simulink model "top_level_arch"  (R2025b)
settings: Solver=VariableStepAuto  StartTime=0.0  StopTime=10.0  RelTol=1e-3
undefined symbols (not defined in the file): D, L
(part 1 of 2)
settings Model: Creator=andgo  LastModifiedBy=andgo

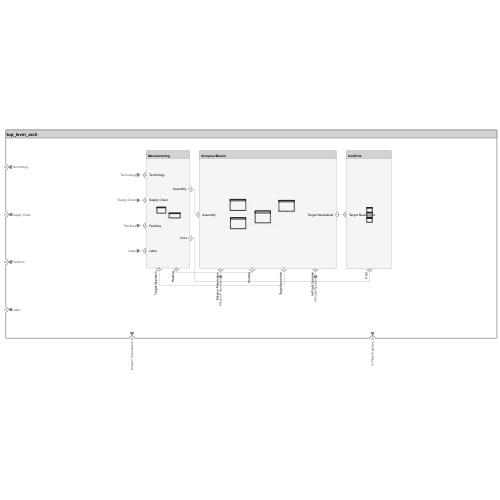
[thumbnail: Simulink's stored preview of the top-level diagram]
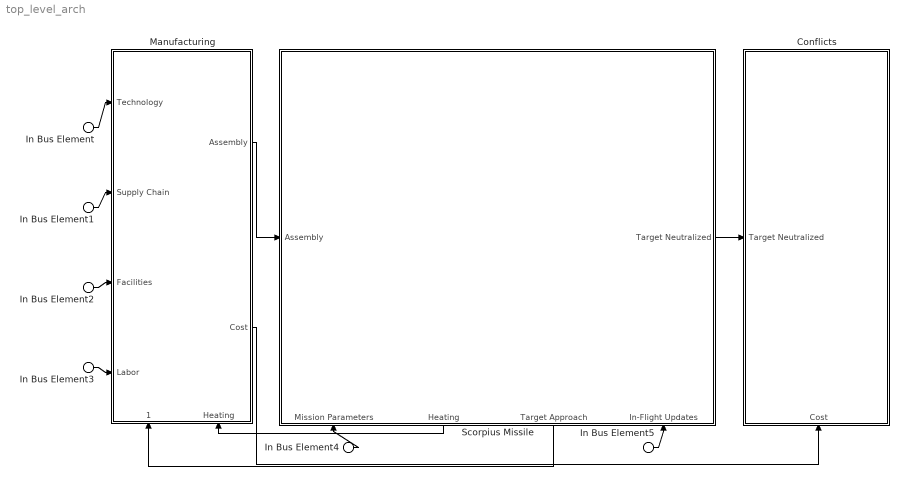
== system top_level_arch ==
  In Bus Element : Inport  PortName=Technology
  In Bus Element1 : Inport  Port=2  PortName=Supply Chain
  In Bus Element2 : Inport  Port=3  PortName=Facilities
  In Bus Element3 : Inport  Port=4  PortName=Labor
  In Bus Element4 : Inport  Port=5  PortName=Mission Parameters
  In Bus Element5 : Inport  Port=6  PortName=In-Flight Updates
  Conflicts : Subsystem
      settings: PortSchema="{\"entries\":[{\"content\":{\"headerSize\":26,\"margin\":15,\"minimumSpacing\":25,\"sides\":[{\"content\":{\"connectorIds\":[\"In2\"]},\"type\":\"ConnectorPlacement.EquallySpacedRectSide\",\"uuid\":\"acffec25-5f7e-46a6-bfc3-7ef631e1638e\"},{\"content\":{\"side\":\"RIGHT\"},\"type\":\"ConnectorPlacement.EquallySpacedRectSide\",\"uuid\":\"2e9e2c31-11a0-4694-98ae-75af4a65f270\"},{\"content\":{\"side\":\"TOP\"},\"type\":\"ConnectorPlacement.EquallySpacedRectSide\",\"uuid\":\"496cd80b-0660-4c9b-9e86-ee3459eee66e\"},{\"content\":{\"connectorIds\":[\"In1\"],\"side\":\"BOTTOM\"},\"type\":\"ConnectorPlacement.EquallySpacedRectSide\",\"uuid\":\"28484b37-6b41-41f8-9797-a09ef52b9345\"}]},\"type\":\"ConnectorPlacement.EquallySpacedConnector\",\"uuid\":\"b09bcaf7-bc67-4c5f-bdb5-a74881794e47\"}],\"packageUris\":[\"http://schema.mathworks.com/mf0/Connector/R2020b\"],\"version\":\"1.0\"}"
  "Manufacturing " : Subsystem
      settings: PortSchema="{\"entries\":[{\"content\":{\"headerSize\":26,\"margin\":15,\"minimumSpacing\":25,\"sides\":[{\"content\":{\"connectorIds\":[\"In3\",\"In4\",\"In5\",\"In6\"]},\"type\":\"ConnectorPlacement.EquallySpacedRectSide\",\"uuid\":\"acffec25-5f7e-46a6-bfc3-7ef631e1638e\"},{\"content\":{\"connectorIds\":[\"Out1\",\"Out2\"],\"side\":\"RIGHT\"},\"type\":\"ConnectorPlacement.EquallySpacedRectSide\",\"uuid\":\"2e9e2c31-11a0-4694-98ae-75af4a65f270\"},{\"content\":{\"side\":\"TOP\"},\"type\":\"ConnectorPlacement.EquallySpacedRectSide\",\"uuid\":\"496cd80b-0660-4c9b-9e86-ee3459eee66e\"},{\"content\":{\"connectorIds\":[\"In1\",\"In2\"],\"side\":\"BOTTOM\"},\"type\":\"ConnectorPlacement.EquallySpacedRectSide\",\"uuid\":\"33532b3b-2f4b-483d-9516-7c4914e8cb27\"}]},\"type\":\"ConnectorPlacement.EquallySpacedConnector\",\"uuid\":\"b09bcaf7-bc67-4c5f-bdb5-a74881794e47\"}],\"packageUris\":[\"http://schema.mathworks.com/mf0/Connector/R2020b\"],\"version\":\"1.0\"}"
  Scorpius Missile : Subsystem
      settings: PortSchema="{\"entries\":[{\"content\":{\"headerSize\":26,\"margin\":15,\"minimumSpacing\":25,\"sides\":[{\"content\":{\"connectorIds\":[\"In3\"]},\"type\":\"ConnectorPlacement.EquallySpacedRectSide\",\"uuid\":\"acffec25-5f7e-46a6-bfc3-7ef631e1638e\"},{\"content\":{\"connectorIds\":[\"Out3\"],\"side\":\"RIGHT\"},\"type\":\"ConnectorPlacement.EquallySpacedRectSide\",\"uuid\":\"2e9e2c31-11a0-4694-98ae-75af4a65f270\"},{\"content\":{\"side\":\"TOP\"},\"type\":\"ConnectorPlacement.EquallySpacedRectSide\",\"uuid\":\"496cd80b-0660-4c9b-9e86-ee3459eee66e\"},{\"content\":{\"connectorIds\":[\"In1\",\"Out1\",\"Out2\",\"In2\"],\"side\":\"BOTTOM\"},\"type\":\"ConnectorPlacement.EquallySpacedRectSide\",\"uuid\":\"f0cf9de3-dec7-4c3c-836d-f09237c2a5d9\"}]},\"type\":\"ConnectorPlacement.EquallySpacedConnector\",\"uuid\":\"b09bcaf7-bc67-4c5f-bdb5-a74881794e47\"}],\"packageUris\":[\"http://schema.mathworks.com/mf0/Connector/R2020b\"],\"version\":\"1.0\"}"
  wires:
  Scorpius Missile/3(Target Neutralized) -> Conflicts/2(Target Neutralized)
  "Manufacturing "/1(Assembly) -> Scorpius Missile/3(Assembly)
  In Bus Element/1 -> "Manufacturing "/3(Technology)
  In Bus Element1/1 -> "Manufacturing "/4(Supply Chain)
  In Bus Element2/1 -> "Manufacturing "/5(Facilities)
  In Bus Element3/1 -> "Manufacturing "/6(Labor)
  In Bus Element4/1 -> Scorpius Missile/1(Mission Parameters)
  In Bus Element5/1 -> Scorpius Missile/2(In-Flight Updates)
  Scorpius Missile/1(Heating) -> "Manufacturing "/2(Heating)
  Scorpius Missile/2(Target Approach) -> "Manufacturing "/1(Target Approach)
  "Manufacturing "/2(Cost) -> Conflicts/1(Cost)

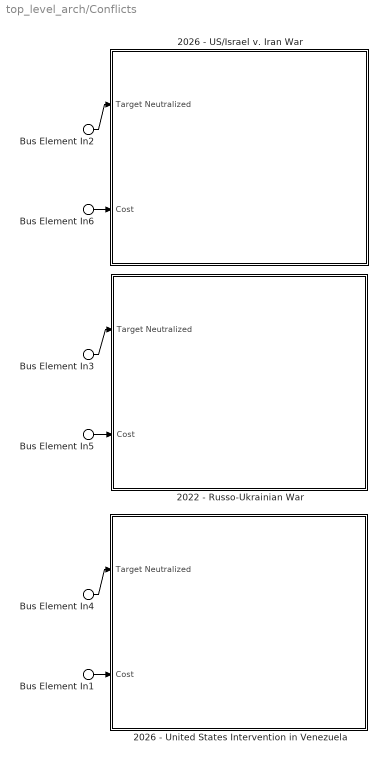
== system top_level_arch/Conflicts ==
  Bus Element In1 : Inport  PortName=Cost
  Bus Element In5 : Inport  PortName=Cost
  Bus Element In6 : Inport  PortName=Cost
  Bus Element In2 : Inport  Port=2  PortName=Target Neutralized
  Bus Element In3 : Inport  Port=2  PortName=Target Neutralized
  Bus Element In4 : Inport  Port=2  PortName=Target Neutralized
  2022 - Russo-Ukrainian War : Subsystem
      settings: PortSchema="{\"entries\":[{\"content\":{\"headerSize\":26,\"margin\":15,\"minimumSpacing\":25,\"sides\":[{\"content\":{\"connectorIds\":[\"In1\",\"In2\"]},\"type\":\"ConnectorPlacement.EquallySpacedRectSide\",\"uuid\":\"acffec25-5f7e-46a6-bfc3-7ef631e1638e\"},{\"content\":{\"side\":\"RIGHT\"},\"type\":\"ConnectorPlacement.EquallySpacedRectSide\",\"uuid\":\"2e9e2c31-11a0-4694-98ae-75af4a65f270\"},{\"content\":{\"side\":\"TOP\"},\"type\":\"ConnectorPlacement.EquallySpacedRectSide\",\"uuid\":\"496cd80b-0660-4c9b-9e86-ee3459eee66e\"}]},\"type\":\"ConnectorPlacement.EquallySpacedConnector\",\"uuid\":\"b09bcaf7-bc67-4c5f-bdb5-a74881794e47\"}],\"packageUris\":[\"http://schema.mathworks.com/mf0/Connector/R2020b\"],\"version\":\"1.0\"}"
  2026 - US/Israel v. Iran War : Subsystem
      settings: PortSchema="{\"entries\":[{\"content\":{\"headerSize\":26,\"margin\":15,\"minimumSpacing\":25,\"sides\":[{\"content\":{\"connectorIds\":[\"In1\",\"In2\"]},\"type\":\"ConnectorPlacement.EquallySpacedRectSide\",\"uuid\":\"acffec25-5f7e-46a6-bfc3-7ef631e1638e\"},{\"content\":{\"side\":\"RIGHT\"},\"type\":\"ConnectorPlacement.EquallySpacedRectSide\",\"uuid\":\"2e9e2c31-11a0-4694-98ae-75af4a65f270\"},{\"content\":{\"side\":\"TOP\"},\"type\":\"ConnectorPlacement.EquallySpacedRectSide\",\"uuid\":\"496cd80b-0660-4c9b-9e86-ee3459eee66e\"}]},\"type\":\"ConnectorPlacement.EquallySpacedConnector\",\"uuid\":\"b09bcaf7-bc67-4c5f-bdb5-a74881794e47\"}],\"packageUris\":[\"http://schema.mathworks.com/mf0/Connector/R2020b\"],\"version\":\"1.0\"}"
  2026 - United States Intervention in Venezuela : Subsystem
      settings: PortSchema="{\"entries\":[{\"content\":{\"headerSize\":26,\"margin\":15,\"minimumSpacing\":25,\"sides\":[{\"content\":{\"connectorIds\":[\"In1\",\"In2\"]},\"type\":\"ConnectorPlacement.EquallySpacedRectSide\",\"uuid\":\"acffec25-5f7e-46a6-bfc3-7ef631e1638e\"},{\"content\":{\"side\":\"RIGHT\"},\"type\":\"ConnectorPlacement.EquallySpacedRectSide\",\"uuid\":\"2e9e2c31-11a0-4694-98ae-75af4a65f270\"},{\"content\":{\"side\":\"TOP\"},\"type\":\"ConnectorPlacement.EquallySpacedRectSide\",\"uuid\":\"496cd80b-0660-4c9b-9e86-ee3459eee66e\"}]},\"type\":\"ConnectorPlacement.EquallySpacedConnector\",\"uuid\":\"b09bcaf7-bc67-4c5f-bdb5-a74881794e47\"}],\"packageUris\":[\"http://schema.mathworks.com/mf0/Connector/R2020b\"],\"version\":\"1.0\"}"
  wires:
  Bus Element In2/1 -> 2026 - US/Israel v. Iran War/1(Target Neutralized)
  Bus Element In3/1 -> 2022 - Russo-Ukrainian War/1(Target Neutralized)
  Bus Element In4/1 -> 2026 - United States Intervention in Venezuela/1(Target Neutralized)
  Bus Element In1/1 -> 2026 - United States Intervention in Venezuela/2(Cost)
  Bus Element In5/1 -> 2022 - Russo-Ukrainian War/2(Cost)
  Bus Element In6/1 -> 2026 - US/Israel v. Iran War/2(Cost)

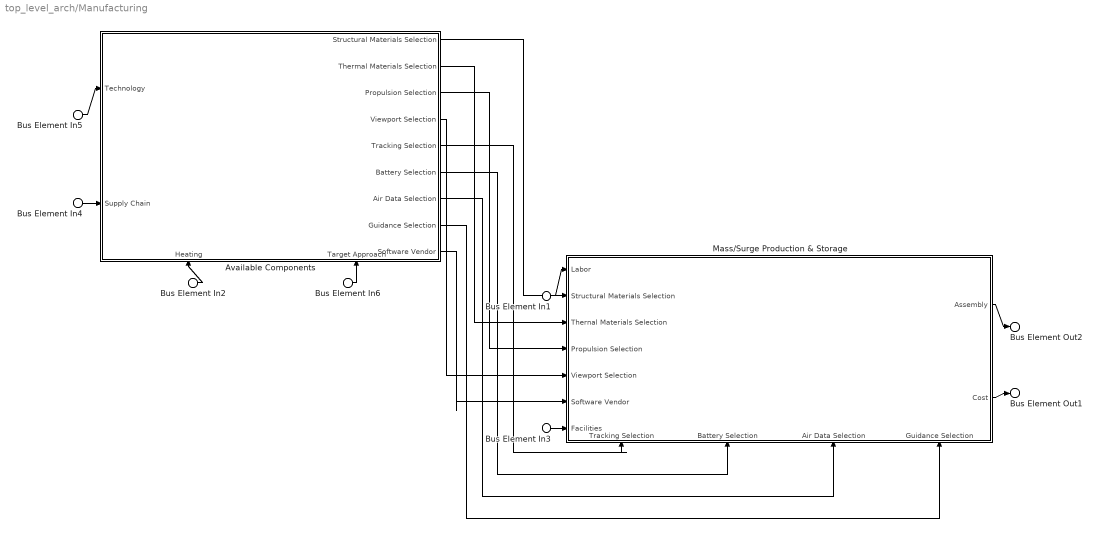
== system top_level_arch/Manufacturing  ==
  Bus Element In6 : Inport  PortName=Target Approach
  Bus Element In2 : Inport  Port=2  PortName=Heating
  Bus Element In5 : Inport  Port=3  PortName=Technology
  Bus Element In4 : Inport  Port=4  PortName=Supply Chain
  Bus Element In3 : Inport  Port=5  PortName=Facilities
  Bus Element In1 : Inport  Port=6  PortName=Labor
  Available Components : Subsystem
      settings: PortSchema="{\"entries\":[{\"content\":{\"headerSize\":26,\"margin\":15,\"minimumSpacing\":25,\"sides\":[{\"content\":{\"connectorIds\":[\"In3\",\"In4\"]},\"type\":\"ConnectorPlacement.EquallySpacedRectSide\",\"uuid\":\"acffec25-5f7e-46a6-bfc3-7ef631e1638e\"},{\"content\":{\"connectorIds\":[\"Out1\",\"Out2\",\"Out3\",\"Out4\",\"Out5\",\"Out6\",\"Out7\",\"Out8\",\"Out9\"],\"side\":\"RIGHT\"},\"type\":\"ConnectorPlacement.EquallySpacedRectSide\",\"uuid\":\"2e9e2c31-11a0-4694-98ae-75af4a65f270\"},{\"content\":{\"side\":\"TOP\"},\"type\":\"ConnectorPlacement.EquallySpacedRectSide\",\"uuid\":\"496cd80b-0660-4c9b-9e86-ee3459eee66e\"},{\"content\":{\"connectorIds\":[\"In1\",\"In2\"],\"side\":\"BOTTOM\"},\"type\":\"ConnectorPlacement.EquallySpacedRectSide\",\"uuid\":\"c248d288-a86e-4b39-8154-69971e55abdb\"}]},\"type\":\"ConnectorPlacement.EquallySpacedConnector\",\"uuid\":\"b09bcaf7-bc67-4c5f-bdb5-a74881794e47\"}],\"packageUris\":[\"http://schema.mathworks.com/mf0/Connector/R2020b\"],\"version\":\"1.0\"}"
  Mass/Surge Production & Storage : Subsystem
      settings: PortSchema="{\"entries\":[{\"content\":{\"headerSize\":26,\"margin\":15,\"minimumSpacing\":25,\"sides\":[{\"content\":{\"connectorIds\":[\"In6\",\"In7\",\"In8\",\"In9\",\"In5\",\"In10\",\"In11\"]},\"type\":\"ConnectorPlacement.EquallySpacedRectSide\",\"uuid\":\"0599d581-e05a-42f2-828a-909155d7b553\"},{\"content\":{\"connectorIds\":[\"Out1\",\"Out2\"],\"side\":\"RIGHT\"},\"type\":\"ConnectorPlacement.EquallySpacedRectSide\",\"uuid\":\"4f3684cd-c181-4c6b-8883-844072d01e34\"},{\"content\":{\"side\":\"TOP\"},\"type\":\"ConnectorPlacement.EquallySpacedRectSide\",\"uuid\":\"71c93445-b4b9-443f-b471-e335a3ed31ea\"},{\"content\":{\"connectorIds\":[\"In1\",\"In2\",\"In3\",\"In4\"],\"side\":\"BOTTOM\"},\"type\":\"ConnectorPlacement.EquallySpacedRectSide\",\"uuid\":\"e60e4bcf-0025-4c31-a0bb-395ca2e6fb9d\"}]},\"type\":\"ConnectorPlacement.EquallySpacedConnector\",\"uuid\":\"086a7661-e694-4344-b95d-ad0347bf3c95\"}],\"packageUris\":[\"http://schema.mathworks.com/mf0/Connector/R2020b\"],\"version\":\"1.0\"}"
  Bus Element Out2 : Outport  PortName=Assembly
  Bus Element Out1 : Outport  Port=2  PortName=Cost
  wires:
  Bus Element In1/1 -> Mass/Surge Production & Storage/6(Labor)
  Bus Element In3/1 -> Mass/Surge Production & Storage/11(Facilities)
  Available Components/1(Structural Materials Selection) -> Mass/Surge Production & Storage/7(Structural Materials Selection)
  Bus Element In5/1 -> Available Components/3(Technology)
  Bus Element In4/1 -> Available Components/4(Supply Chain)
  Mass/Surge Production & Storage/2(Cost) -> Bus Element Out1/1
  Mass/Surge Production & Storage/1(Assembly) -> Bus Element Out2/1
  Available Components/2(Thermal Materials Selection) -> Mass/Surge Production & Storage/8(Thernal Materials Selection)
  Available Components/3(Propulsion Selection) -> Mass/Surge Production & Storage/9(Propulsion Selection)
  Available Components/9(Software Vendor) -> Mass/Surge Production & Storage/10(Software Vendor)
  Available Components/5(Tracking Selection) -> Mass/Surge Production & Storage/1(Tracking Selection)
  Available Components/6(Battery Selection) -> Mass/Surge Production & Storage/2(Battery Selection)
  Available Components/7(Air Data Selection) -> Mass/Surge Production & Storage/3(Air Data Selection)
  Available Components/8(Guidance Selection) -> Mass/Surge Production & Storage/4(Guidance Selection)
  Bus Element In2/1 -> Available Components/1(Heating)
  Bus Element In6/1 -> Available Components/2(Target Approach)
  Available Components/4(Viewport Selection) -> Mass/Surge Production & Storage/5(Viewport Selection)

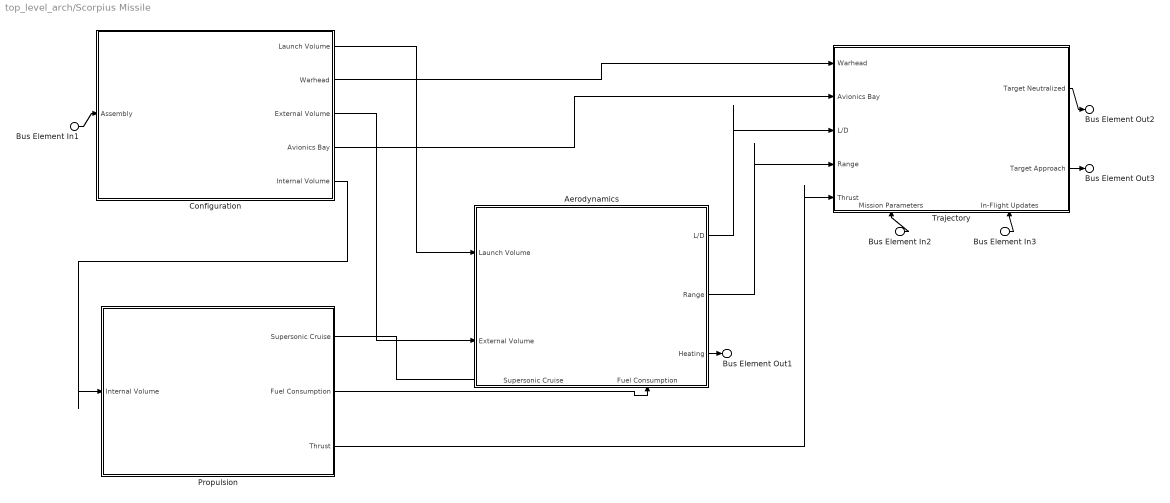
== system top_level_arch/Scorpius Missile ==
  Bus Element In2 : Inport  PortName=Mission Parameters
  Bus Element In3 : Inport  Port=2  PortName=In-Flight Updates
  Bus Element In1 : Inport  Port=3  PortName=Assembly
  Aerodynamics : Subsystem  Variant=on  VariantControlMode=label  LabelModeActiveChoice=true
      settings: PortSchema="{\"entries\":[{\"content\":{\"headerSize\":38,\"margin\":15,\"minimumSpacing\":25,\"sides\":[{\"content\":{\"connectorIds\":[\"In3\",\"In4\"]},\"type\":\"ConnectorPlacement.EquallySpacedRectSide\",\"uuid\":\"5f197e08-86ca-4cb0-8773-2eafa3be5f58\"},{\"content\":{\"connectorIds\":[\"Out2\",\"Out3\",\"Out1\"],\"side\":\"RIGHT\"},\"type\":\"ConnectorPlacement.EquallySpacedRectSide\",\"uuid\":\"8f6035a6-196b-436f-97c5-6c30a28d2ffa\"},{\"content\":{\"side\":\"TOP\"},\"type\":\"ConnectorPlacement.EquallySpacedRectSide\",\"uuid\":\"47fbcf31-f69d-4ec2-89cd-2bc4268e79ee\"},{\"content\":{\"connectorIds\":[\"In1\",\"In2\"],\"side\":\"BOTTOM\"},\"type\":\"ConnectorPlacement.EquallySpacedRectSide\",\"uuid\":\"4028af42-eefe-4e40-a537-59e66f9c77fb\"}]},\"type\":\"ConnectorPlacement.EquallySpacedConnector\",\"uuid\":\"7bd4d14b-9a13-45a8-b2b2-976268dd46fb\"}],\"packageUris\":[\"http://schema.mathworks.com/mf0/Connector/R2020b\"],\"version\":\"1.0\"}"
  Configuration : Subsystem
      settings: PortSchema="{\"entries\":[{\"content\":{\"headerSize\":26,\"margin\":15,\"minimumSpacing\":25,\"sides\":[{\"content\":{\"connectorIds\":[\"In1\"]},\"type\":\"ConnectorPlacement.EquallySpacedRectSide\",\"uuid\":\"32e1f4e9-0392-4c12-9305-55f9b62cf007\"},{\"content\":{\"connectorIds\":[\"Out3\",\"Out2\",\"Out5\",\"Out4\",\"Out1\"],\"side\":\"RIGHT\"},\"type\":\"ConnectorPlacement.EquallySpacedRectSide\",\"uuid\":\"8bf8c952-69c8-496e-947f-24d197d632d3\"},{\"content\":{\"side\":\"TOP\"},\"type\":\"ConnectorPlacement.EquallySpacedRectSide\",\"uuid\":\"adf3e777-baf5-48a6-a5b4-f0ede588bd33\"},{\"content\":{\"side\":\"BOTTOM\"},\"type\":\"ConnectorPlacement.EquallySpacedRectSide\",\"uuid\":\"91d27ee5-9ea1-4b68-a684-98df6014676a\"}]},\"type\":\"ConnectorPlacement.EquallySpacedConnector\",\"uuid\":\"9ec8f034-0877-461e-a570-0bf1a23861f1\"}],\"packageUris\":[\"http://schema.mathworks.com/mf0/Connector/R2020b\"],\"version\":\"1.0\"}"
  Propulsion : Subsystem  Description=|
      | Relevant Trade Study .m file listed in Stereotypes. 
      | Cannot link .m files directly.
      | Other teams encountered this issue as well.
      settings: PortSchema="{\"entries\":[{\"content\":{\"headerSize\":26,\"margin\":15,\"minimumSpacing\":25,\"sides\":[{\"content\":{\"connectorIds\":[\"In1\"]},\"type\":\"ConnectorPlacement.EquallySpacedRectSide\",\"uuid\":\"acffec25-5f7e-46a6-bfc3-7ef631e1638e\"},{\"content\":{\"connectorIds\":[\"Out1\",\"Out2\",\"Out3\"],\"side\":\"RIGHT\"},\"type\":\"ConnectorPlacement.EquallySpacedRectSide\",\"uuid\":\"2e9e2c31-11a0-4694-98ae-75af4a65f270\"},{\"content\":{\"side\":\"TOP\"},\"type\":\"ConnectorPlacement.EquallySpacedRectSide\",\"uuid\":\"496cd80b-0660-4c9b-9e86-ee3459eee66e\"}]},\"type\":\"ConnectorPlacement.EquallySpacedConnector\",\"uuid\":\"b09bcaf7-bc67-4c5f-bdb5-a74881794e47\"}],\"packageUris\":[\"http://schema.mathworks.com/mf0/Connector/R2020b\"],\"version\":\"1.0\"}"
  Trajectory : Subsystem  Description=|
      | Relevant Trade Study .m file listed in Stereotypes. 
      | Cannot link .m files directly.
      | Other teams encountered this issue as well.
      settings: PortSchema="{\"entries\":[{\"content\":{\"headerSize\":26,\"margin\":15,\"minimumSpacing\":25,\"sides\":[{\"content\":{\"connectorIds\":[\"In1\",\"In7\",\"In3\",\"In4\",\"In5\"]},\"type\":\"ConnectorPlacement.EquallySpacedRectSide\",\"uuid\":\"acffec25-5f7e-46a6-bfc3-7ef631e1638e\"},{\"content\":{\"connectorIds\":[\"Out1\",\"Out2\"],\"side\":\"RIGHT\"},\"type\":\"ConnectorPlacement.EquallySpacedRectSide\",\"uuid\":\"2e9e2c31-11a0-4694-98ae-75af4a65f270\"},{\"content\":{\"side\":\"TOP\"},\"type\":\"ConnectorPlacement.EquallySpacedRectSide\",\"uuid\":\"496cd80b-0660-4c9b-9e86-ee3459eee66e\"},{\"content\":{\"connectorIds\":[\"In2\",\"In6\"],\"side\":\"BOTTOM\"},\"type\":\"ConnectorPlacement.EquallySpacedRectSide\",\"uuid\":\"ff4f15f2-78c9-4b4d-8b3c-eee51a6070cf\"}]},\"type\":\"ConnectorPlacement.EquallySpacedConnector\",\"uuid\":\"b09bcaf7-bc67-4c5f-bdb5-a74881794e47\"}],\"packageUris\":[\"http://schema.mathworks.com/mf0/Connector/R2020b\"],\"version\":\"1.0\"}"
  Bus Element Out1 : Outport  PortName=Heating
  Bus Element Out3 : Outport  Port=2  PortName=Target Approach
  Bus Element Out2 : Outport  Port=3  PortName=Target Neutralized
  wires:
  Bus Element In1/1 -> Configuration/1(Assembly)
  Configuration/4(Avionics Bay) -> Trajectory/7(Avionics Bay)
  Bus Element In2/1 -> Trajectory/2(Mission Parameters)
  Bus Element In3/1 -> Trajectory/6(In-Flight Updates)
  Configuration/1(Internal Volume) -> Propulsion/1(Internal Volume)
  Configuration/5(External Volume) -> Aerodynamics/4(External Volume)
  Configuration/3(Launch Volume) -> Aerodynamics/3(Launch Volume)
  Propulsion/1(Supersonic Cruise) -> Aerodynamics/1(Supersonic Cruise)
  Propulsion/2(Fuel Consumption) -> Aerodynamics/2(Fuel Consumption)
  Aerodynamics/2(L/D) -> Trajectory/3(L/D)
  Aerodynamics/3(Range) -> Trajectory/4(Range)
  Trajectory/1(Target Neutralized) -> Bus Element Out2/1
  Aerodynamics/1(Heating) -> Bus Element Out1/1
  Trajectory/2(Target Approach) -> Bus Element Out3/1
  Propulsion/3(Thrust) -> Trajectory/5(Thrust)
  Configuration/2(Warhead) -> Trajectory/1(Warhead)

== system top_level_arch/Conflicts/2022 - Russo-Ukrainian War ==
  Bus Element In1 : Inport  PortName=Target Neutralized
  Bus Element In2 : Inport  Port=2  PortName=Cost

== system top_level_arch/Conflicts/2026 - US//Israel v. Iran War ==
  Bus Element In1 : Inport  PortName=Target Neutralized
  Bus Element In2 : Inport  Port=2  PortName=Cost

== system top_level_arch/Conflicts/2026 - United States Intervention in Venezuela ==
  Bus Element In1 : Inport  PortName=Target Neutralized
  Bus Element In2 : Inport  Port=2  PortName=Cost

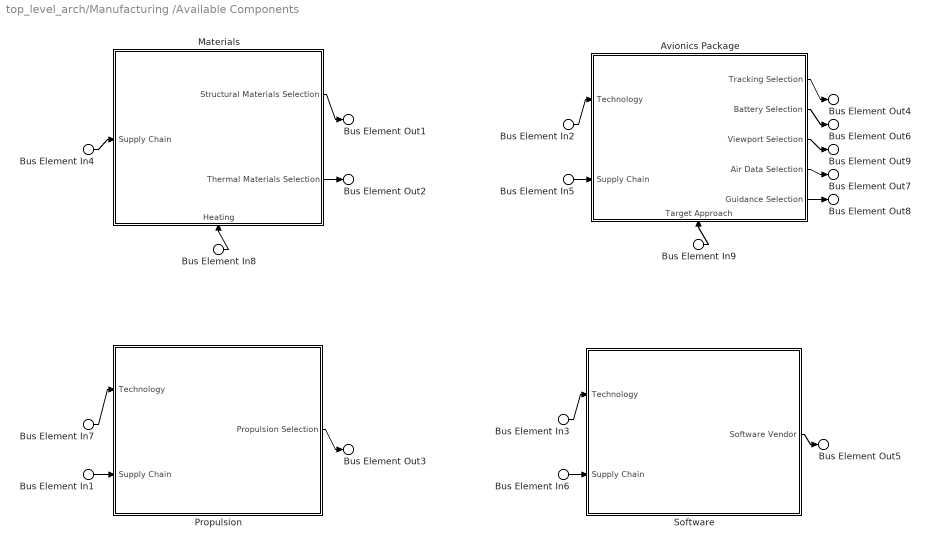
== system top_level_arch/Manufacturing /Available Components ==
  Bus Element In8 : Inport  PortName=Heating
  Bus Element In9 : Inport  Port=2  PortName=Target Approach
  Bus Element In2 : Inport  Port=3  PortName=Technology
  Bus Element In3 : Inport  Port=3  PortName=Technology
  Bus Element In7 : Inport  Port=3  PortName=Technology
  Bus Element In{1,4..6} (4 alike) : Inport  Port=4  PortName=Supply Chain
  Avionics Package : Subsystem
      settings: PortSchema="{\"entries\":[{\"content\":{\"headerSize\":26,\"margin\":15,\"minimumSpacing\":25,\"sides\":[{\"content\":{\"connectorIds\":[\"In2\",\"In3\"]},\"type\":\"ConnectorPlacement.EquallySpacedRectSide\",\"uuid\":\"acffec25-5f7e-46a6-bfc3-7ef631e1638e\"},{\"content\":{\"connectorIds\":[\"Out1\",\"Out2\",\"Out3\",\"Out4\",\"Out5\"],\"side\":\"RIGHT\"},\"type\":\"ConnectorPlacement.EquallySpacedRectSide\",\"uuid\":\"2e9e2c31-11a0-4694-98ae-75af4a65f270\"},{\"content\":{\"side\":\"TOP\"},\"type\":\"ConnectorPlacement.EquallySpacedRectSide\",\"uuid\":\"496cd80b-0660-4c9b-9e86-ee3459eee66e\"},{\"content\":{\"connectorIds\":[\"In1\"],\"side\":\"BOTTOM\"},\"type\":\"ConnectorPlacement.EquallySpacedRectSide\",\"uuid\":\"3c8f2b30-ca4f-4a07-a307-f07a27b8cebe\"}]},\"type\":\"ConnectorPlacement.EquallySpacedConnector\",\"uuid\":\"b09bcaf7-bc67-4c5f-bdb5-a74881794e47\"}],\"packageUris\":[\"http://schema.mathworks.com/mf0/Connector/R2020b\"],\"version\":\"1.0\"}"
  Materials : Subsystem
      settings: PortSchema="{\"entries\":[{\"content\":{\"headerSize\":26,\"margin\":15,\"minimumSpacing\":25,\"sides\":[{\"content\":{\"connectorIds\":[\"In2\"]},\"type\":\"ConnectorPlacement.EquallySpacedRectSide\",\"uuid\":\"32e1f4e9-0392-4c12-9305-55f9b62cf007\"},{\"content\":{\"connectorIds\":[\"Out1\",\"Out2\"],\"side\":\"RIGHT\"},\"type\":\"ConnectorPlacement.EquallySpacedRectSide\",\"uuid\":\"8bf8c952-69c8-496e-947f-24d197d632d3\"},{\"content\":{\"side\":\"TOP\"},\"type\":\"ConnectorPlacement.EquallySpacedRectSide\",\"uuid\":\"adf3e777-baf5-48a6-a5b4-f0ede588bd33\"},{\"content\":{\"connectorIds\":[\"In1\"],\"side\":\"BOTTOM\"},\"type\":\"ConnectorPlacement.EquallySpacedRectSide\",\"uuid\":\"078485eb-bf6f-42cf-8a3e-170b8ee8b571\"}]},\"type\":\"ConnectorPlacement.EquallySpacedConnector\",\"uuid\":\"9ec8f034-0877-461e-a570-0bf1a23861f1\"}],\"packageUris\":[\"http://schema.mathworks.com/mf0/Connector/R2020b\"],\"version\":\"1.0\"}"
  Propulsion : Subsystem  Variant=on  VariantControlMode=label  LabelModeActiveChoice=true
      settings: PortSchema="{\"entries\":[{\"content\":{\"headerSize\":38,\"margin\":15,\"minimumSpacing\":25,\"sides\":[{\"content\":{\"connectorIds\":[\"In1\",\"In2\"]},\"type\":\"ConnectorPlacement.EquallySpacedRectSide\",\"uuid\":\"6bf547dd-331a-449e-ac23-c58fb11a97ac\"},{\"content\":{\"connectorIds\":[\"Out1\"],\"side\":\"RIGHT\"},\"type\":\"ConnectorPlacement.EquallySpacedRectSide\",\"uuid\":\"fd538850-fa48-484a-8745-4b783330bf7c\"},{\"content\":{\"side\":\"TOP\"},\"type\":\"ConnectorPlacement.EquallySpacedRectSide\",\"uuid\":\"f77f67e7-993d-4952-a6b8-f4e06992afc3\"}]},\"type\":\"ConnectorPlacement.EquallySpacedConnector\",\"uuid\":\"84bbcc3e-e353-48cf-9125-7f316d0ada6d\"}],\"packageUris\":[\"http://schema.mathworks.com/mf0/Connector/R2020b\"],\"version\":\"1.0\"}"
  Software : Subsystem
      settings: PortSchema="{\"entries\":[{\"content\":{\"headerSize\":26,\"margin\":15,\"minimumSpacing\":25,\"sides\":[{\"content\":{\"connectorIds\":[\"In1\",\"In2\"]},\"type\":\"ConnectorPlacement.EquallySpacedRectSide\",\"uuid\":\"acffec25-5f7e-46a6-bfc3-7ef631e1638e\"},{\"content\":{\"connectorIds\":[\"Out1\"],\"side\":\"RIGHT\"},\"type\":\"ConnectorPlacement.EquallySpacedRectSide\",\"uuid\":\"2e9e2c31-11a0-4694-98ae-75af4a65f270\"},{\"content\":{\"side\":\"TOP\"},\"type\":\"ConnectorPlacement.EquallySpacedRectSide\",\"uuid\":\"496cd80b-0660-4c9b-9e86-ee3459eee66e\"}]},\"type\":\"ConnectorPlacement.EquallySpacedConnector\",\"uuid\":\"b09bcaf7-bc67-4c5f-bdb5-a74881794e47\"}],\"packageUris\":[\"http://schema.mathworks.com/mf0/Connector/R2020b\"],\"version\":\"1.0\"}"
  Bus Element Out1 : Outport  PortName=Structural Materials Selection
  Bus Element Out2 : Outport  Port=2  PortName=Thermal Materials Selection
  Bus Element Out3 : Outport  Port=3  PortName=Propulsion Selection
  Bus Element Out9 : Outport  Port=4  PortName=Viewport Selection
  Bus Element Out4 : Outport  Port=5  PortName=Tracking Selection
  Bus Element Out6 : Outport  Port=6  PortName=Battery Selection
  Bus Element Out7 : Outport  Port=7  PortName=Air Data Selection
  Bus Element Out8 : Outport  Port=8  PortName=Guidance Selection
  Bus Element Out5 : Outport  Port=9  PortName=Software Vendor
  wires:
  Bus Element In2/1 -> Avionics Package/2(Technology)
  Bus Element In3/1 -> Software/1(Technology)
  Bus Element In4/1 -> Materials/2(Supply Chain)
  Bus Element In5/1 -> Avionics Package/3(Supply Chain)
  Bus Element In6/1 -> Software/2(Supply Chain)
  Bus Element In1/1 -> Propulsion/2(Supply Chain)
  Bus Element In7/1 -> Propulsion/1(Technology)
  Materials/1(Structural Materials Selection) -> Bus Element Out1/1
  Materials/2(Thermal Materials Selection) -> Bus Element Out2/1
  Propulsion/1(Propulsion Selection) -> Bus Element Out3/1
  Software/1(Software Vendor) -> Bus Element Out5/1
  Avionics Package/1(Tracking Selection) -> Bus Element Out4/1
  Avionics Package/2(Battery Selection) -> Bus Element Out6/1
  Avionics Package/4(Air Data Selection) -> Bus Element Out7/1
  Avionics Package/5(Guidance Selection) -> Bus Element Out8/1
  Bus Element In8/1 -> Materials/1(Heating)
  Bus Element In9/1 -> Avionics Package/1(Target Approach)
  Avionics Package/3(Viewport Selection) -> Bus Element Out9/1

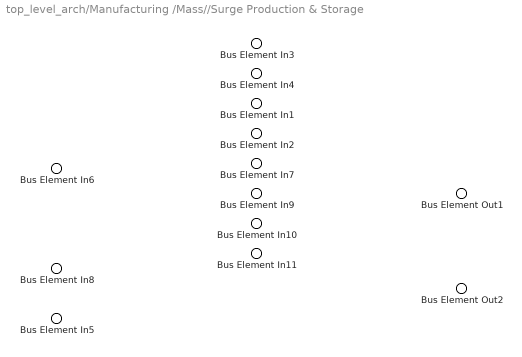
== system top_level_arch/Manufacturing /Mass//Surge Production & Storage ==
  Bus Element In1 : Inport  PortName=Tracking Selection
  Bus Element In7 : Inport  Port=2  PortName=Battery Selection
  Bus Element In9 : Inport  Port=3  PortName=Air Data Selection
  Bus Element In10 : Inport  Port=4  PortName=Guidance Selection
  Bus Element In11 : Inport  Port=5  PortName=Viewport Selection
  Bus Element In5 : Inport  Port=6  PortName=Labor
  Bus Element In6 : Inport  Port=7  PortName=Structural Materials Selection
  Bus Element In3 : Inport  Port=8  PortName=Thernal Materials Selection
  Bus Element In4 : Inport  Port=9  PortName=Propulsion Selection
  Bus Element In2 : Inport  Port=10  PortName=Software Vendor
  Bus Element In8 : Inport  Port=11  PortName=Facilities
  Bus Element Out1 : Outport  PortName=Assembly
  Bus Element Out2 : Outport  Port=2  PortName=Cost

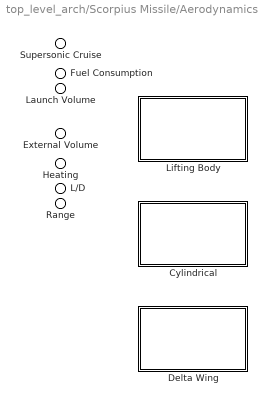
== system top_level_arch/Scorpius Missile/Aerodynamics ==
  Supersonic Cruise : Inport
  Fuel Consumption : Inport  Port=2
  Launch Volume : Inport  Port=3
  External Volume : Inport  Port=4
  Cylindrical : Subsystem  VariantControl=false
      settings: PortSchema="{\"entries\":[{\"content\":{\"headerSize\":26,\"margin\":15,\"minimumSpacing\":25,\"sides\":[{\"content\":{},\"type\":\"ConnectorPlacement.EquallySpacedRectSide\",\"uuid\":\"ac629711-1768-428b-8fd7-79e4fe2b35a1\"},{\"content\":{\"side\":\"RIGHT\"},\"type\":\"ConnectorPlacement.EquallySpacedRectSide\",\"uuid\":\"b9c43ceb-249f-4c48-950c-a08a709e2313\"},{\"content\":{\"side\":\"TOP\"},\"type\":\"ConnectorPlacement.EquallySpacedRectSide\",\"uuid\":\"78a92a70-2dde-432d-9083-f129ee7bb076\"}]},\"type\":\"ConnectorPlacement.EquallySpacedConnector\",\"uuid\":\"b2b722ac-28c2-40e7-82d5-b0c5abc634fd\"}],\"packageUris\":[\"http://schema.mathworks.com/mf0/Connector/R2020b\"],\"version\":\"1.0\"}"
  Delta Wing : Subsystem  VariantControl=Cylindrical1
      settings: PortSchema="{\"entries\":[{\"content\":{\"headerSize\":26,\"margin\":15,\"minimumSpacing\":25,\"sides\":[{\"content\":{},\"type\":\"ConnectorPlacement.EquallySpacedRectSide\",\"uuid\":\"ac629711-1768-428b-8fd7-79e4fe2b35a1\"},{\"content\":{\"side\":\"RIGHT\"},\"type\":\"ConnectorPlacement.EquallySpacedRectSide\",\"uuid\":\"b9c43ceb-249f-4c48-950c-a08a709e2313\"},{\"content\":{\"side\":\"TOP\"},\"type\":\"ConnectorPlacement.EquallySpacedRectSide\",\"uuid\":\"78a92a70-2dde-432d-9083-f129ee7bb076\"}]},\"type\":\"ConnectorPlacement.EquallySpacedConnector\",\"uuid\":\"b2b722ac-28c2-40e7-82d5-b0c5abc634fd\"}],\"packageUris\":[\"http://schema.mathworks.com/mf0/Connector/R2020b\"],\"version\":\"1.0\"}"
  Lifting Body : Subsystem  VariantControl=true  mask{L_D=[]}
      settings: PortSchema="{\"entries\":[{\"content\":{\"headerSize\":26,\"margin\":15,\"minimumSpacing\":25,\"sides\":[{\"content\":{},\"type\":\"ConnectorPlacement.EquallySpacedRectSide\",\"uuid\":\"ac629711-1768-428b-8fd7-79e4fe2b35a1\"},{\"content\":{\"side\":\"RIGHT\"},\"type\":\"ConnectorPlacement.EquallySpacedRectSide\",\"uuid\":\"b9c43ceb-249f-4c48-950c-a08a709e2313\"},{\"content\":{\"side\":\"TOP\"},\"type\":\"ConnectorPlacement.EquallySpacedRectSide\",\"uuid\":\"78a92a70-2dde-432d-9083-f129ee7bb076\"}]},\"type\":\"ConnectorPlacement.EquallySpacedConnector\",\"uuid\":\"b2b722ac-28c2-40e7-82d5-b0c5abc634fd\"}],\"packageUris\":[\"http://schema.mathworks.com/mf0/Connector/R2020b\"],\"version\":\"1.0\"}"
  Heating : Outport
  L/D : Outport  Port=2
  Range : Outport  Port=3

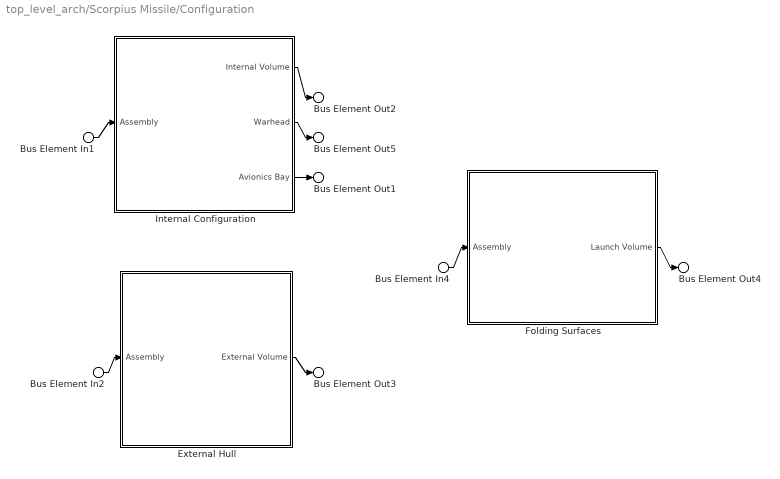
== system top_level_arch/Scorpius Missile/Configuration ==
  Bus Element In1 : Inport  PortName=Assembly
  Bus Element In2 : Inport  PortName=Assembly
  Bus Element In4 : Inport  PortName=Assembly
  External Hull : Subsystem
      settings: PortSchema="{\"entries\":[{\"content\":{\"headerSize\":26,\"margin\":15,\"minimumSpacing\":25,\"sides\":[{\"content\":{\"connectorIds\":[\"In1\"]},\"type\":\"ConnectorPlacement.EquallySpacedRectSide\",\"uuid\":\"32e1f4e9-0392-4c12-9305-55f9b62cf007\"},{\"content\":{\"connectorIds\":[\"Out1\"],\"side\":\"RIGHT\"},\"type\":\"ConnectorPlacement.EquallySpacedRectSide\",\"uuid\":\"8bf8c952-69c8-496e-947f-24d197d632d3\"},{\"content\":{\"side\":\"TOP\"},\"type\":\"ConnectorPlacement.EquallySpacedRectSide\",\"uuid\":\"adf3e777-baf5-48a6-a5b4-f0ede588bd33\"}]},\"type\":\"ConnectorPlacement.EquallySpacedConnector\",\"uuid\":\"9ec8f034-0877-461e-a570-0bf1a23861f1\"}],\"packageUris\":[\"http://schema.mathworks.com/mf0/Connector/R2020b\"],\"version\":\"1.0\"}"
  Folding Surfaces : Subsystem  Variant=on  VariantControlMode=label  LabelModeActiveChoice=true
      settings: PortSchema="{\"entries\":[{\"content\":{\"headerSize\":38,\"margin\":15,\"minimumSpacing\":25,\"sides\":[{\"content\":{\"connectorIds\":[\"In1\"]},\"type\":\"ConnectorPlacement.EquallySpacedRectSide\",\"uuid\":\"5f197e08-86ca-4cb0-8773-2eafa3be5f58\"},{\"content\":{\"connectorIds\":[\"Out1\"],\"side\":\"RIGHT\"},\"type\":\"ConnectorPlacement.EquallySpacedRectSide\",\"uuid\":\"8f6035a6-196b-436f-97c5-6c30a28d2ffa\"},{\"content\":{\"side\":\"TOP\"},\"type\":\"ConnectorPlacement.EquallySpacedRectSide\",\"uuid\":\"47fbcf31-f69d-4ec2-89cd-2bc4268e79ee\"}]},\"type\":\"ConnectorPlacement.EquallySpacedConnector\",\"uuid\":\"7bd4d14b-9a13-45a8-b2b2-976268dd46fb\"}],\"packageUris\":[\"http://schema.mathworks.com/mf0/Connector/R2020b\"],\"version\":\"1.0\"}"
  Internal Configuration : Subsystem  Description=|
      | Relevant Trade Study .m file listed in Stereotypes. 
      | Cannot link .m files directly.
      | Other teams encountered this issue as well.
      settings: PortSchema="{\"entries\":[{\"content\":{\"headerSize\":26,\"margin\":15,\"minimumSpacing\":25,\"sides\":[{\"content\":{\"connectorIds\":[\"In1\"]},\"type\":\"ConnectorPlacement.EquallySpacedRectSide\",\"uuid\":\"32e1f4e9-0392-4c12-9305-55f9b62cf007\"},{\"content\":{\"connectorIds\":[\"Out1\",\"Out2\",\"Out3\"],\"side\":\"RIGHT\"},\"type\":\"ConnectorPlacement.EquallySpacedRectSide\",\"uuid\":\"8bf8c952-69c8-496e-947f-24d197d632d3\"},{\"content\":{\"side\":\"TOP\"},\"type\":\"ConnectorPlacement.EquallySpacedRectSide\",\"uuid\":\"adf3e777-baf5-48a6-a5b4-f0ede588bd33\"}]},\"type\":\"ConnectorPlacement.EquallySpacedConnector\",\"uuid\":\"9ec8f034-0877-461e-a570-0bf1a23861f1\"}],\"packageUris\":[\"http://schema.mathworks.com/mf0/Connector/R2020b\"],\"version\":\"1.0\"}"
  Bus Element Out2 : Outport  PortName=Internal Volume
  Bus Element Out5 : Outport  Port=2  PortName=Warhead
  Bus Element Out4 : Outport  Port=3  PortName=Launch Volume
  Bus Element Out1 : Outport  Port=4  PortName=Avionics Bay
  Bus Element Out3 : Outport  Port=5  PortName=External Volume
  wires:
  Bus Element In1/1 -> Internal Configuration/1(Assembly)
  Bus Element In2/1 -> External Hull/1(Assembly)
  Internal Configuration/1(Internal Volume) -> Bus Element Out2/1
  External Hull/1(External Volume) -> Bus Element Out3/1
  Internal Configuration/3(Avionics Bay) -> Bus Element Out1/1
  Internal Configuration/2(Warhead) -> Bus Element Out5/1
  Bus Element In4/1 -> Folding Surfaces/1(Assembly)
  Folding Surfaces/1(Launch Volume) -> Bus Element Out4/1

== system top_level_arch/Scorpius Missile/Propulsion ==
  Bus Element In1 : Inport  PortName=Internal Volume
  Fuel/Oxidizer Tank : Subsystem
      settings: PortSchema="{\"entries\":[{\"content\":{\"headerSize\":26,\"margin\":15,\"minimumSpacing\":25,\"sides\":[{\"content\":{\"connectorIds\":[\"In1\"]},\"type\":\"ConnectorPlacement.EquallySpacedRectSide\",\"uuid\":\"f725402c-10b5-4b82-85cc-51bef2710ba8\"},{\"content\":{\"connectorIds\":[\"Out1\"],\"side\":\"RIGHT\"},\"type\":\"ConnectorPlacement.EquallySpacedRectSide\",\"uuid\":\"62fc519a-e2d1-4367-b68f-022d97ba9f16\"},{\"content\":{\"side\":\"TOP\"},\"type\":\"ConnectorPlacement.EquallySpacedRectSide\",\"uuid\":\"613b120d-3cdc-496e-8a51-984c64e3d49e\"}]},\"type\":\"ConnectorPlacement.EquallySpacedConnector\",\"uuid\":\"aaea6f75-d808-4e3f-996d-2fe6c7697c49\"}],\"packageUris\":[\"http://schema.mathworks.com/mf0/Connector/R2020b\"],\"version\":\"1.0\"}"
  RDRE : Subsystem  mask{Thrust=[]}
      settings: PortSchema="{\"entries\":[{\"content\":{\"headerSize\":26,\"margin\":15,\"minimumSpacing\":25,\"sides\":[{\"content\":{\"connectorIds\":[\"In1\"]},\"type\":\"ConnectorPlacement.EquallySpacedRectSide\",\"uuid\":\"f725402c-10b5-4b82-85cc-51bef2710ba8\"},{\"content\":{\"connectorIds\":[\"Out1\",\"Out2\",\"Out3\"],\"side\":\"RIGHT\"},\"type\":\"ConnectorPlacement.EquallySpacedRectSide\",\"uuid\":\"62fc519a-e2d1-4367-b68f-022d97ba9f16\"},{\"content\":{\"side\":\"TOP\"},\"type\":\"ConnectorPlacement.EquallySpacedRectSide\",\"uuid\":\"613b120d-3cdc-496e-8a51-984c64e3d49e\"}]},\"type\":\"ConnectorPlacement.EquallySpacedConnector\",\"uuid\":\"aaea6f75-d808-4e3f-996d-2fe6c7697c49\"}],\"packageUris\":[\"http://schema.mathworks.com/mf0/Connector/R2020b\"],\"version\":\"1.0\"}"
  Bus Element Out1 : Outport  PortName=Supersonic Cruise
  Bus Element Out3 : Outport  Port=2  PortName=Fuel Consumption
  Bus Element Out2 : Outport  Port=3  PortName=Thrust
  wires:
  Bus Element In1/1 -> Fuel/Oxidizer Tank/1(Internal Volume)
  Fuel/Oxidizer Tank/1(Fuel Capacity) -> RDRE/1(Fuel Capacity)
  RDRE/2(Fuel Consumption) -> Bus Element Out3/1
  RDRE/1(Supersonic Cruise) -> Bus Element Out1/1
  RDRE/3(Thrust) -> Bus Element Out2/1

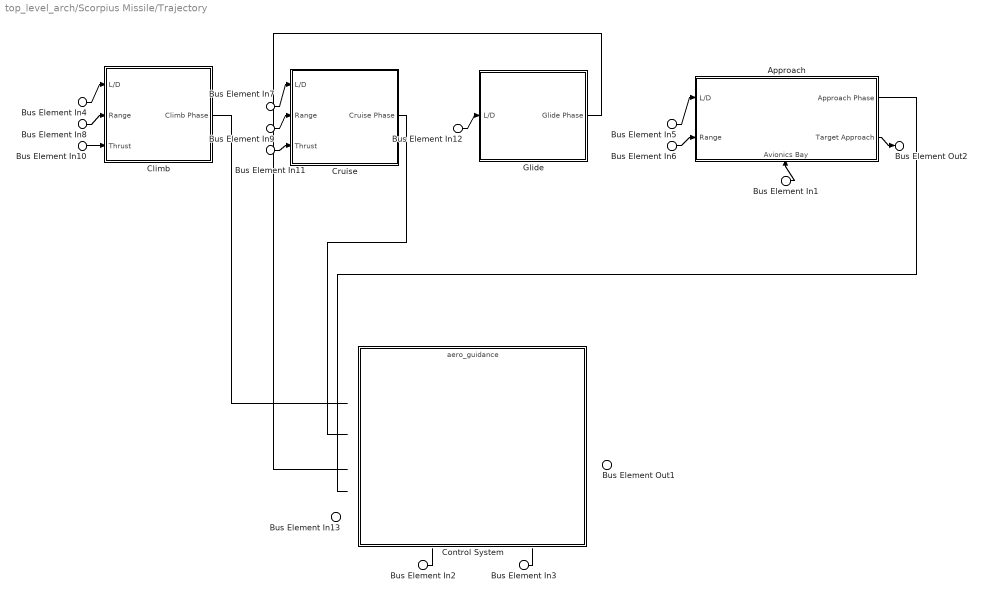
== system top_level_arch/Scorpius Missile/Trajectory ==
  Bus Element In13 : Inport  PortName=Warhead
  Bus Element In2 : Inport  Port=2  PortName=Mission Parameters
  Bus Element In{4..5,7,12} (4 alike) : Inport  Port=3  PortName=L/D
  Bus Element In6 : Inport  Port=4  PortName=Range
  Bus Element In8 : Inport  Port=4  PortName=Range
  Bus Element In9 : Inport  Port=4  PortName=Range
  Bus Element In10 : Inport  Port=5  PortName=Thrust
  Bus Element In11 : Inport  Port=5  PortName=Thrust
  Bus Element In3 : Inport  Port=6  PortName=In-Flight Updates
  Bus Element In1 : Inport  Port=7  PortName=Avionics Bay
  Approach : Subsystem  Variant=on  VariantControlMode=label  LabelModeActiveChoice=true
      settings: PortSchema="{\"entries\":[{\"content\":{\"headerSize\":38,\"margin\":15,\"minimumSpacing\":25,\"sides\":[{\"content\":{\"connectorIds\":[\"In2\",\"In3\"]},\"type\":\"ConnectorPlacement.EquallySpacedRectSide\",\"uuid\":\"5f197e08-86ca-4cb0-8773-2eafa3be5f58\"},{\"content\":{\"connectorIds\":[\"Out1\",\"Out2\"],\"side\":\"RIGHT\"},\"type\":\"ConnectorPlacement.EquallySpacedRectSide\",\"uuid\":\"8f6035a6-196b-436f-97c5-6c30a28d2ffa\"},{\"content\":{\"side\":\"TOP\"},\"type\":\"ConnectorPlacement.EquallySpacedRectSide\",\"uuid\":\"47fbcf31-f69d-4ec2-89cd-2bc4268e79ee\"},{\"content\":{\"connectorIds\":[\"In1\"],\"side\":\"BOTTOM\"},\"type\":\"ConnectorPlacement.EquallySpacedRectSide\",\"uuid\":\"7584f524-88c9-4ef7-88fb-252bdf179e00\"}]},\"type\":\"ConnectorPlacement.EquallySpacedConnector\",\"uuid\":\"7bd4d14b-9a13-45a8-b2b2-976268dd46fb\"}],\"packageUris\":[\"http://schema.mathworks.com/mf0/Connector/R2020b\"],\"version\":\"1.0\"}"
  Climb : Subsystem  Description=|
      | Relevant Trade Study .m file listed in Stereotypes. 
      | Cannot link .m files directly.
      | Other teams encountered this issue as well.
      settings: PortSchema="{\"entries\":[{\"content\":{\"headerSize\":26,\"margin\":15,\"minimumSpacing\":25,\"sides\":[{\"content\":{\"connectorIds\":[\"In1\",\"In2\",\"In3\"]},\"type\":\"ConnectorPlacement.EquallySpacedRectSide\",\"uuid\":\"f725402c-10b5-4b82-85cc-51bef2710ba8\"},{\"content\":{\"connectorIds\":[\"Out1\"],\"side\":\"RIGHT\"},\"type\":\"ConnectorPlacement.EquallySpacedRectSide\",\"uuid\":\"62fc519a-e2d1-4367-b68f-022d97ba9f16\"},{\"content\":{\"side\":\"TOP\"},\"type\":\"ConnectorPlacement.EquallySpacedRectSide\",\"uuid\":\"613b120d-3cdc-496e-8a51-984c64e3d49e\"}]},\"type\":\"ConnectorPlacement.EquallySpacedConnector\",\"uuid\":\"aaea6f75-d808-4e3f-996d-2fe6c7697c49\"}],\"packageUris\":[\"http://schema.mathworks.com/mf0/Connector/R2020b\"],\"version\":\"1.0\"}"
  Control System : ModelReference  ModelNameDialog=aero_guidance  SimulationMode=Normal  ModelReferenceVersion=11.4
      settings: PortSchema="{\"entries\":[{\"content\":{\"headerSize\":38,\"margin\":15,\"minimumSpacing\":25,\"sides\":[{\"content\":{},\"type\":\"ConnectorPlacement.EquallySpacedRectSide\",\"uuid\":\"f725402c-10b5-4b82-85cc-51bef2710ba8\"},{\"content\":{\"side\":\"RIGHT\"},\"type\":\"ConnectorPlacement.EquallySpacedRectSide\",\"uuid\":\"62fc519a-e2d1-4367-b68f-022d97ba9f16\"},{\"content\":{\"side\":\"TOP\"},\"type\":\"ConnectorPlacement.EquallySpacedRectSide\",\"uuid\":\"613b120d-3cdc-496e-8a51-984c64e3d49e\"},{\"content\":{\"side\":\"BOTTOM\"},\"type\":\"ConnectorPlacement.EquallySpacedRectSide\",\"uuid\":\"35a5b99a-36dd-4c19-a137-7e7534f66045\"}]},\"type\":\"ConnectorPlacement.EquallySpacedConnector\",\"uuid\":\"aaea6f75-d808-4e3f-996d-2fe6c7697c49\"}],\"packageUris\":[\"http://schema.mathworks.com/mf0/Connector/R2020b\"],\"version\":\"1.0\"}"
  Cruise : Subsystem  Description=|
      | Relevant Trade Study .m file listed in Stereotypes. 
      | Cannot link .m files directly.
      | Other teams encountered this issue as well.
      settings: PortSchema="{\"entries\":[{\"content\":{\"headerSize\":26,\"margin\":15,\"minimumSpacing\":25,\"sides\":[{\"content\":{\"connectorIds\":[\"In1\",\"In2\",\"In3\"]},\"type\":\"ConnectorPlacement.EquallySpacedRectSide\",\"uuid\":\"f725402c-10b5-4b82-85cc-51bef2710ba8\"},{\"content\":{\"connectorIds\":[\"Out1\"],\"side\":\"RIGHT\"},\"type\":\"ConnectorPlacement.EquallySpacedRectSide\",\"uuid\":\"62fc519a-e2d1-4367-b68f-022d97ba9f16\"},{\"content\":{\"side\":\"TOP\"},\"type\":\"ConnectorPlacement.EquallySpacedRectSide\",\"uuid\":\"613b120d-3cdc-496e-8a51-984c64e3d49e\"}]},\"type\":\"ConnectorPlacement.EquallySpacedConnector\",\"uuid\":\"aaea6f75-d808-4e3f-996d-2fe6c7697c49\"}],\"packageUris\":[\"http://schema.mathworks.com/mf0/Connector/R2020b\"],\"version\":\"1.0\"}"
  Glide : Subsystem
      settings: PortSchema="{\"entries\":[{\"content\":{\"headerSize\":26,\"margin\":15,\"minimumSpacing\":25,\"sides\":[{\"content\":{\"connectorIds\":[\"In1\"]},\"type\":\"ConnectorPlacement.EquallySpacedRectSide\",\"uuid\":\"f725402c-10b5-4b82-85cc-51bef2710ba8\"},{\"content\":{\"connectorIds\":[\"Out1\"],\"side\":\"RIGHT\"},\"type\":\"ConnectorPlacement.EquallySpacedRectSide\",\"uuid\":\"62fc519a-e2d1-4367-b68f-022d97ba9f16\"},{\"content\":{\"side\":\"TOP\"},\"type\":\"ConnectorPlacement.EquallySpacedRectSide\",\"uuid\":\"613b120d-3cdc-496e-8a51-984c64e3d49e\"}]},\"type\":\"ConnectorPlacement.EquallySpacedConnector\",\"uuid\":\"aaea6f75-d808-4e3f-996d-2fe6c7697c49\"}],\"packageUris\":[\"http://schema.mathworks.com/mf0/Connector/R2020b\"],\"version\":\"1.0\"}"
  Bus Element Out1 : Outport  PortName=Target Neutralized
  Bus Element Out2 : Outport  Port=2  PortName=Target Approach
  wires:
  Bus Element In5/1 -> Approach/2(L/D)
  Bus Element In6/1 -> Approach/3(Range)
  Approach/2(Target Approach) -> Bus Element Out2/1
  Bus Element In1/1 -> Approach/1(Avionics Bay)
  Bus Element In4/1 -> Climb/1(L/D)
  Bus Element In7/1 -> Cruise/1(L/D)
  Bus Element In8/1 -> Climb/2(Range)
  Bus Element In9/1 -> Cruise/2(Range)
  Bus Element In10/1 -> Climb/3(Thrust)
  Bus Element In11/1 -> Cruise/3(Thrust)
  Bus Element In12/1 -> Glide/1(L/D)
  Climb/1(Climb Phase) -> ?
  Cruise/1(Cruise Phase) -> ?
  Glide/1(Glide Phase) -> ?
  Approach/1(Approach Phase) -> ?
  Bus Element In2/1 -> ?
  Bus Element In3/1 -> ?
  ? -> Bus Element Out1/1

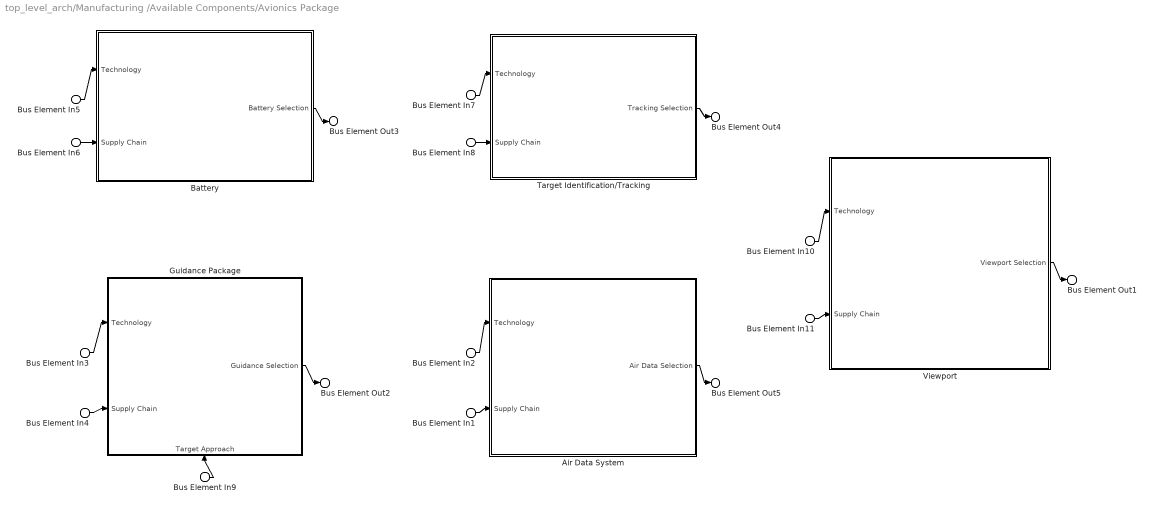
== system top_level_arch/Manufacturing /Available Components/Avionics Package ==
  Bus Element In9 : Inport  PortName=Target Approach
  Bus Element In{2..3,5,7,10} (5 alike) : Inport  Port=2  PortName=Technology
  Bus Element In{1,4,6,8,11} (5 alike) : Inport  Port=3  PortName=Supply Chain
  Air Data System : Subsystem  Variant=on  VariantControlMode=label  LabelModeActiveChoice=true
      settings: PortSchema="{\"entries\":[{\"content\":{\"headerSize\":38,\"margin\":15,\"minimumSpacing\":25,\"sides\":[{\"content\":{\"connectorIds\":[\"In1\",\"In2\"]},\"type\":\"ConnectorPlacement.EquallySpacedRectSide\",\"uuid\":\"5f197e08-86ca-4cb0-8773-2eafa3be5f58\"},{\"content\":{\"connectorIds\":[\"Out1\"],\"side\":\"RIGHT\"},\"type\":\"ConnectorPlacement.EquallySpacedRectSide\",\"uuid\":\"8f6035a6-196b-436f-97c5-6c30a28d2ffa\"},{\"content\":{\"side\":\"TOP\"},\"type\":\"ConnectorPlacement.EquallySpacedRectSide\",\"uuid\":\"47fbcf31-f69d-4ec2-89cd-2bc4268e79ee\"}]},\"type\":\"ConnectorPlacement.EquallySpacedConnector\",\"uuid\":\"7bd4d14b-9a13-45a8-b2b2-976268dd46fb\"}],\"packageUris\":[\"http://schema.mathworks.com/mf0/Connector/R2020b\"],\"version\":\"1.0\"}"
  Battery : Subsystem  Variant=on  VariantControlMode=label  LabelModeActiveChoice=true
      settings: PortSchema="{\"entries\":[{\"content\":{\"headerSize\":38,\"margin\":15,\"minimumSpacing\":25,\"sides\":[{\"content\":{\"connectorIds\":[\"In1\",\"In2\"]},\"type\":\"ConnectorPlacement.EquallySpacedRectSide\",\"uuid\":\"5f197e08-86ca-4cb0-8773-2eafa3be5f58\"},{\"content\":{\"connectorIds\":[\"Out1\"],\"side\":\"RIGHT\"},\"type\":\"ConnectorPlacement.EquallySpacedRectSide\",\"uuid\":\"8f6035a6-196b-436f-97c5-6c30a28d2ffa\"},{\"content\":{\"side\":\"TOP\"},\"type\":\"ConnectorPlacement.EquallySpacedRectSide\",\"uuid\":\"47fbcf31-f69d-4ec2-89cd-2bc4268e79ee\"}]},\"type\":\"ConnectorPlacement.EquallySpacedConnector\",\"uuid\":\"7bd4d14b-9a13-45a8-b2b2-976268dd46fb\"}],\"packageUris\":[\"http://schema.mathworks.com/mf0/Connector/R2020b\"],\"version\":\"1.0\"}"
  Guidance Package : Subsystem  Variant=on  VariantControlMode=label  LabelModeActiveChoice=true
      settings: PortSchema="{\"entries\":[{\"content\":{\"headerSize\":38,\"margin\":15,\"minimumSpacing\":25,\"sides\":[{\"content\":{\"connectorIds\":[\"In2\",\"In3\"]},\"type\":\"ConnectorPlacement.EquallySpacedRectSide\",\"uuid\":\"5f197e08-86ca-4cb0-8773-2eafa3be5f58\"},{\"content\":{\"connectorIds\":[\"Out1\"],\"side\":\"RIGHT\"},\"type\":\"ConnectorPlacement.EquallySpacedRectSide\",\"uuid\":\"8f6035a6-196b-436f-97c5-6c30a28d2ffa\"},{\"content\":{\"side\":\"TOP\"},\"type\":\"ConnectorPlacement.EquallySpacedRectSide\",\"uuid\":\"47fbcf31-f69d-4ec2-89cd-2bc4268e79ee\"},{\"content\":{\"connectorIds\":[\"In1\"],\"side\":\"BOTTOM\"},\"type\":\"ConnectorPlacement.EquallySpacedRectSide\",\"uuid\":\"b11169f0-5fd7-4830-a46f-2a114b8ae254\"}]},\"type\":\"ConnectorPlacement.EquallySpacedConnector\",\"uuid\":\"7bd4d14b-9a13-45a8-b2b2-976268dd46fb\"}],\"packageUris\":[\"http://schema.mathworks.com/mf0/Connector/R2020b\"],\"version\":\"1.0\"}"
  Target Identification/Tracking : Subsystem
      settings: PortSchema="{\"entries\":[{\"content\":{\"headerSize\":26,\"margin\":15,\"minimumSpacing\":25,\"sides\":[{\"content\":{\"connectorIds\":[\"In1\",\"In2\"]},\"type\":\"ConnectorPlacement.EquallySpacedRectSide\",\"uuid\":\"acffec25-5f7e-46a6-bfc3-7ef631e1638e\"},{\"content\":{\"connectorIds\":[\"Out1\"],\"side\":\"RIGHT\"},\"type\":\"ConnectorPlacement.EquallySpacedRectSide\",\"uuid\":\"2e9e2c31-11a0-4694-98ae-75af4a65f270\"},{\"content\":{\"side\":\"TOP\"},\"type\":\"ConnectorPlacement.EquallySpacedRectSide\",\"uuid\":\"496cd80b-0660-4c9b-9e86-ee3459eee66e\"}]},\"type\":\"ConnectorPlacement.EquallySpacedConnector\",\"uuid\":\"b09bcaf7-bc67-4c5f-bdb5-a74881794e47\"}],\"packageUris\":[\"http://schema.mathworks.com/mf0/Connector/R2020b\"],\"version\":\"1.0\"}"
  Viewport : Subsystem  Variant=on  VariantControlMode=label  LabelModeActiveChoice=true
      settings: PortSchema="{\"entries\":[{\"content\":{\"headerSize\":38,\"margin\":15,\"minimumSpacing\":25,\"sides\":[{\"content\":{\"connectorIds\":[\"In1\",\"In2\"]},\"type\":\"ConnectorPlacement.EquallySpacedRectSide\",\"uuid\":\"70986375-b72e-4108-b911-41ca64153cab\"},{\"content\":{\"connectorIds\":[\"Out1\"],\"side\":\"RIGHT\"},\"type\":\"ConnectorPlacement.EquallySpacedRectSide\",\"uuid\":\"d221f7c6-182a-4ade-be54-ac418ac64639\"},{\"content\":{\"side\":\"TOP\"},\"type\":\"ConnectorPlacement.EquallySpacedRectSide\",\"uuid\":\"a83e170a-9f73-4a8d-b534-7ec6dccb39d7\"}]},\"type\":\"ConnectorPlacement.EquallySpacedConnector\",\"uuid\":\"a1b51bcc-6139-40e2-b668-fd8dff97de78\"}],\"packageUris\":[\"http://schema.mathworks.com/mf0/Connector/R2020b\"],\"version\":\"1.0\"}"
  Bus Element Out4 : Outport  PortName=Tracking Selection
  Bus Element Out3 : Outport  Port=2  PortName=Battery Selection
  Bus Element Out1 : Outport  Port=3  PortName=Viewport Selection
  Bus Element Out5 : Outport  Port=4  PortName=Air Data Selection
  Bus Element Out2 : Outport  Port=5  PortName=Guidance Selection
  wires:
  Bus Element In3/1 -> Guidance Package/2(Technology)
  Bus Element In4/1 -> Guidance Package/3(Supply Chain)
  Guidance Package/1(Guidance Selection) -> Bus Element Out2/1
  Bus Element In5/1 -> Battery/1(Technology)
  Bus Element In6/1 -> Battery/2(Supply Chain)
  Battery/1(Battery Selection) -> Bus Element Out3/1
  Bus Element In1/1 -> Air Data System/2(Supply Chain)
  Bus Element In2/1 -> Air Data System/1(Technology)
  Bus Element In7/1 -> Target Identification/Tracking/1(Technology)
  Bus Element In8/1 -> Target Identification/Tracking/2(Supply Chain)
  Target Identification/Tracking/1(Tracking Selection) -> Bus Element Out4/1
  Air Data System/1(Air Data Selection) -> Bus Element Out5/1
  Bus Element In9/1 -> Guidance Package/1(Target Approach)
  Bus Element In10/1 -> Viewport/1(Technology)
  Bus Element In11/1 -> Viewport/2(Supply Chain)
  Viewport/1(Viewport Selection) -> Bus Element Out1/1

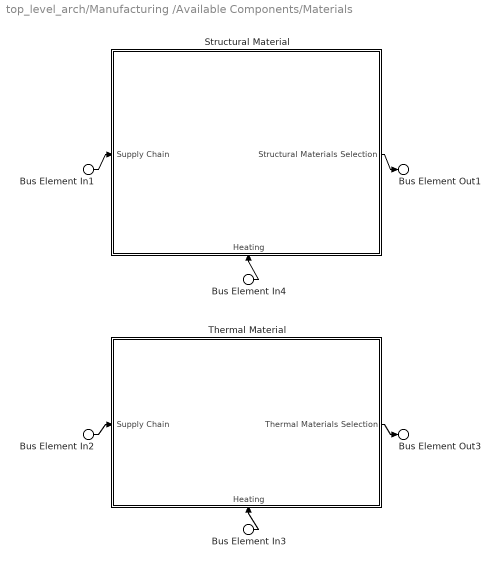
== system top_level_arch/Manufacturing /Available Components/Materials ==
  Bus Element In3 : Inport  PortName=Heating
  Bus Element In4 : Inport  PortName=Heating
  Bus Element In1 : Inport  Port=2  PortName=Supply Chain
  Bus Element In2 : Inport  Port=2  PortName=Supply Chain
  Structural Material : Subsystem  Variant=on  VariantControlMode=label  LabelModeActiveChoice=true
      settings: PortSchema="{\"entries\":[{\"content\":{\"headerSize\":38,\"margin\":15,\"minimumSpacing\":25,\"sides\":[{\"content\":{\"connectorIds\":[\"In2\"]},\"type\":\"ConnectorPlacement.EquallySpacedRectSide\",\"uuid\":\"6bf547dd-331a-449e-ac23-c58fb11a97ac\"},{\"content\":{\"connectorIds\":[\"Out1\"],\"side\":\"RIGHT\"},\"type\":\"ConnectorPlacement.EquallySpacedRectSide\",\"uuid\":\"fd538850-fa48-484a-8745-4b783330bf7c\"},{\"content\":{\"side\":\"TOP\"},\"type\":\"ConnectorPlacement.EquallySpacedRectSide\",\"uuid\":\"f77f67e7-993d-4952-a6b8-f4e06992afc3\"},{\"content\":{\"connectorIds\":[\"In1\"],\"side\":\"BOTTOM\"},\"type\":\"ConnectorPlacement.EquallySpacedRectSide\",\"uuid\":\"9b2a486f-9227-4c81-9238-4dfdc16b5c38\"}]},\"type\":\"ConnectorPlacement.EquallySpacedConnector\",\"uuid\":\"84bbcc3e-e353-48cf-9125-7f316d0ada6d\"}],\"packageUris\":[\"http://schema.mathworks.com/mf0/Connector/R2020b\"],\"version\":\"1.0\"}"
  Thermal Material : Subsystem
      settings: PortSchema="{\"entries\":[{\"content\":{\"headerSize\":26,\"margin\":15,\"minimumSpacing\":25,\"sides\":[{\"content\":{\"connectorIds\":[\"In2\"]},\"type\":\"ConnectorPlacement.EquallySpacedRectSide\",\"uuid\":\"32e1f4e9-0392-4c12-9305-55f9b62cf007\"},{\"content\":{\"connectorIds\":[\"Out1\"],\"side\":\"RIGHT\"},\"type\":\"ConnectorPlacement.EquallySpacedRectSide\",\"uuid\":\"8bf8c952-69c8-496e-947f-24d197d632d3\"},{\"content\":{\"side\":\"TOP\"},\"type\":\"ConnectorPlacement.EquallySpacedRectSide\",\"uuid\":\"adf3e777-baf5-48a6-a5b4-f0ede588bd33\"},{\"content\":{\"connectorIds\":[\"In1\"],\"side\":\"BOTTOM\"},\"type\":\"ConnectorPlacement.EquallySpacedRectSide\",\"uuid\":\"d8d00ec3-61e5-4885-9c41-be6e4afbdcb5\"}]},\"type\":\"ConnectorPlacement.EquallySpacedConnector\",\"uuid\":\"9ec8f034-0877-461e-a570-0bf1a23861f1\"}],\"packageUris\":[\"http://schema.mathworks.com/mf0/Connector/R2020b\"],\"version\":\"1.0\"}"
  Bus Element Out1 : Outport  PortName=Structural Materials Selection
  Bus Element Out3 : Outport  Port=2  PortName=Thermal Materials Selection
  wires:
  Bus Element In1/1 -> Structural Material/2(Supply Chain)
  Bus Element In2/1 -> Thermal Material/2(Supply Chain)
  Structural Material/1(Structural Materials Selection) -> Bus Element Out1/1
  Thermal Material/1(Thermal Materials Selection) -> Bus Element Out3/1
  Bus Element In3/1 -> Thermal Material/1(Heating)
  Bus Element In4/1 -> Structural Material/1(Heating)
